simulink model "untitled2"  (R2013b)
settings: Solver=ode45  StartTime=0.0  StopTime=10.0  RelTol=1e-3
settings Model: Creator=mwegiere  LastModifiedBy=mwegiere

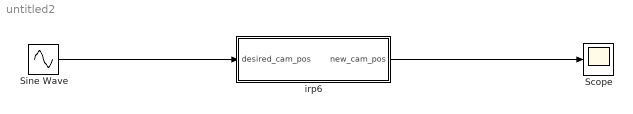
== system untitled2 ==
  Scope : Scope
  Sine Wave : Sin  Amplitude=10  Frequency=0.1  SampleTime=0
  irp6 : Subsystem
  wires:
  Sine Wave/1 -> irp6/1("desired_cam_pos ")
  irp6/1("new_cam_pos ") -> Scope/1

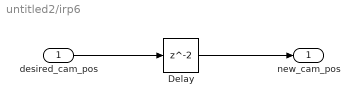
== system untitled2/irp6 ==
  "desired_cam_pos " : Inport
  Delay : Delay  InitialCondition=0
  "new_cam_pos " : Outport
  wires:
  "desired_cam_pos "/1 -> Delay/1
  Delay/1 -> "new_cam_pos "/1
